simulink model "input_shaping_ei"  (R2023a)
settings: configuration reference "config" (kept outside this file)
model workspace (MATLAB code in the model file):
  | cmdLim = Simulink.Parameter;
  | cmdLim.Value = 15;
  | cmdLim.Description = 'Limit for controlling the maximum surface command angle.';
  | cmdLim.Min = 0;
  | cmdLim.Max = 90;
  | cmdLim.DocUnits = 'deg';
  | 
  | dispGain = Simulink.Parameter;
  | dispGain.Value = 0.75;
  | dispGain.Description = 'Gain applied to the displacement error.';
  | dispGain.Min = 0;
  | dispGain.Max = [];
  | dispGain.DocUnits = 'deg/sec/deg';
  | 
  | dispLim = Simulink.Parameter;
  | dispLim.Value = 30;
  | dispLim.Description = 'Limit for controlling the maximum commanded angle.';
  | dispLim.Min = 0;
  | dispLim.Max = 180;
  | dispLim.DocUnits = 'deg';
  | 
  | intGain = Simulink.Parameter;
  | intGain.Value = 0.5;
  | intGain.Description = 'Gain applied to the integral error.';
  | intGain.Min = 0;
  | intGain.Max = [];
  | intGain.DocUnits = 'deg/sec/deg/sec';
  | 
  | intLim = Simulink.Parameter;
  | intLim.Value = 5;
  | intLim.Description = 'Limit for controlling the maximum commanded angle.';
  | intLim.Min = 0;
  | intLim.Max = 90;
  | intLim.DocUnits = 'deg';
  | 
  | rateGain = Simulink.Parameter;
  | rateGain.Value = 2;
  | rateGain.Description = 'Gain applied to the rate error.';
  | rateGain.Min = 0;
  | rateGain.Max = [];
  | rateGain.DocUnits = 'deg/deg/sec';
  | 
  | rateLim = Simulink.Parameter;
  | rateLim.Value = 6;
  | rateLim.Description = 'Limit for controlling the maximum commanded angle.';
  | rateLim.Min = 0;
  | rateLim.Max = 180;
  | rateLim.DocUnits = 'deg/sec';
  | 
  | hdgGain = Simulink.Parameter;
  | hdgGain.Value = 0.015;
settings Model: RequirementInfo={} %GIDa_fe9045fd_0412_4b6e_8206_617cc20e6fde  DataDictionary=model_config.sldd  Creator=Administrator  LastModifiedBy=Administrator
settings ConfigSetRef: SourceName=config

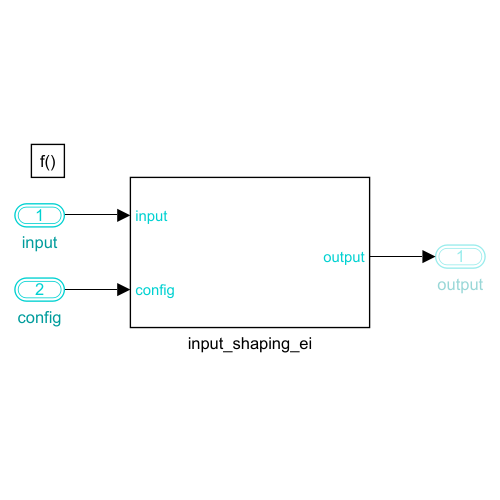
[thumbnail: Simulink's stored preview of the top-level diagram]
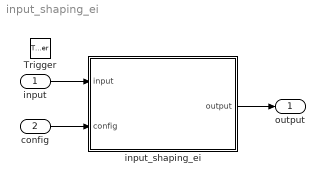
== system input_shaping_ei ==
  input : Inport  OutDataTypeStr=Bus: InputShapingInput  BusOutputAsStruct=on
  config : Inport  Port=2  OutDataTypeStr=Bus: InputShapingConfig  BusOutputAsStruct=on
  Trigger : TriggerPort  TriggerType=function-call  VariantControl=(inherit)  PortDimensions=1
  input_shaping_ei : Subsystem  SystemSampleTime=10e-5
  output : Outport  OutDataTypeStr=Bus: InputShapingOutput  BusOutputAsStruct=on
      settings: EnsureOutportIsVirtual=on
  wires:
  input/1 -> input_shaping_ei/1(input)
  config/1 -> input_shaping_ei/2(config)
  input_shaping_ei/1(output) -> output/1

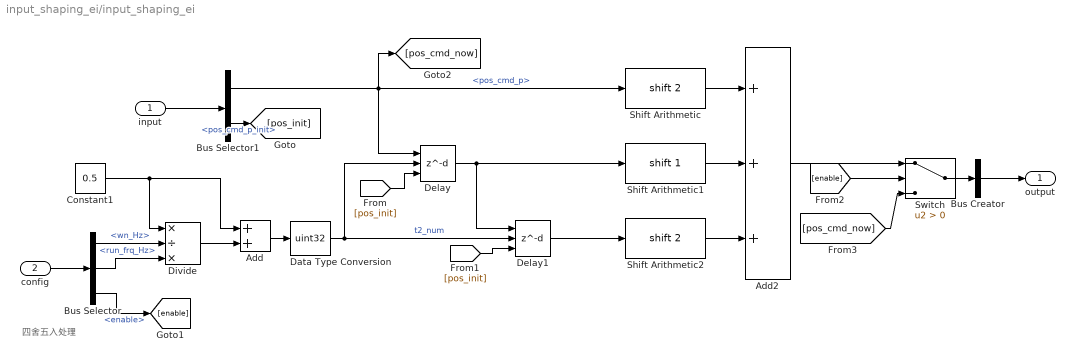
== system input_shaping_ei/input_shaping_ei ==
  note: 四舍五入处理
  input : Inport  OutDataTypeStr=Bus: InputShapingInput
  config : Inport  Port=2  OutDataTypeStr=Bus: InputShapingConfig
  Add : Sum
  Add2 : Sum  Inputs=+++
  Bus Creator : BusCreator  Inputs=1  OutDataTypeStr=Bus: InputShapingOutput  NonVirtualBus=on
      settings: InheritFromInputs=off
  Bus Selector : BusSelector  OutputSignals=wn_Hz,run_frq_Hz,enable
  Bus Selector1 : BusSelector  OutputSignals=pos_cmd_p,pos_cmd_p_init
  Constant1 : Constant  Value=0.5  OutDataTypeStr=single
  Data Type Conversion : DataTypeConversion  OutDataTypeStr=uint32  SaturateOnIntegerOverflow=off  RndMeth=Floor
  Delay : Delay  DelayLengthSource=Input port  DelayLengthUpperLimit=500  InitialConditionSource=Input port  UseCircularBuffer=on  StateName=t2_delay_buffer
      settings: InputPortMap=u0,p1,p4
  Delay1 : Delay  DelayLengthSource=Input port  DelayLengthUpperLimit=500  InitialConditionSource=Input port  UseCircularBuffer=on  StateName=t3_delay_buffer
      settings: InputPortMap=u0,p1,p4
  Divide : Product  Inputs=*/*
  Shift Arithmetic : ArithShift  BitShiftNumber=2
  Shift Arithmetic1 : ArithShift  BitShiftNumber=1
  Shift Arithmetic2 : ArithShift  BitShiftNumber=2
  Switch : Switch  Criteria=u2 > Threshold  SaturateOnIntegerOverflow=off  InputSameDT=off
  output : Outport  OutDataTypeStr=Bus: InputShapingOutput
  wires:
  Bus Selector/1 -> Divide/2  "<wn_Hz>"
  config/1 -> Bus Selector/1
  Constant1/1 -> Add/1, Divide/1
  Bus Selector1/1 -> [pos_cmd_now], Delay/1, Shift Arithmetic/1  "<pos_cmd_p>"
  Delay/1 -> Delay1/1, Shift Arithmetic1/1
  Bus Selector/2 -> Divide/3  "<run_frq_Hz>"
  Add/1 -> Data Type Conversion/1
  Divide/1 -> Add/2
  input/1 -> Bus Selector1/1
  Data Type Conversion/1 -> Delay1/2, Delay/2  "t2_num"
  Shift Arithmetic1/1 -> Add2/2
  Delay1/1 -> Shift Arithmetic2/1
  Shift Arithmetic/1 -> Add2/1
  Shift Arithmetic2/1 -> Add2/3
  Bus Creator/1 -> output/1
  Bus Selector1/2 -> [pos_init]  "<pos_cmd_p_init>"
  [pos_init] -> Delay/3
  [pos_init] -> Delay1/3
  Bus Selector/3 -> [enable]  "<enable>"
  [enable] -> Switch/2
  Add2/1 -> Switch/1
  Switch/1 -> Bus Creator/1
  [pos_cmd_now] -> Switch/3
